simulink model "projeto_2016"  (R2016a)
settings: Solver=VariableStepAuto  StartTime=0.0  StopTime=t_sim  MaxStep=passo_integracao  RelTol=1e-3
values from neighbouring files (symbols this model uses):
  Kat = .3    (= 0.3)    [geracao.m]    (also in geracao_quadrado.m; parametros.m)
  x1_0 = -pi    (= -3.14159265359)    [geracao.m]    (also in geracao_quadrado.m = 0; parametros.m = 0)
  x2_0 = 0    [geracao.m]    (also in geracao_quadrado.m; parametros.m)
  x3_0 = 0    [geracao.m]    (also in geracao_quadrado.m; parametros.m)
  x4_0 = 0    [geracao.m]    (also in geracao_quadrado.m; parametros.m)
settings Model: Creator=ivanp_o3t94tg  LastModifiedBy=ivan_prog

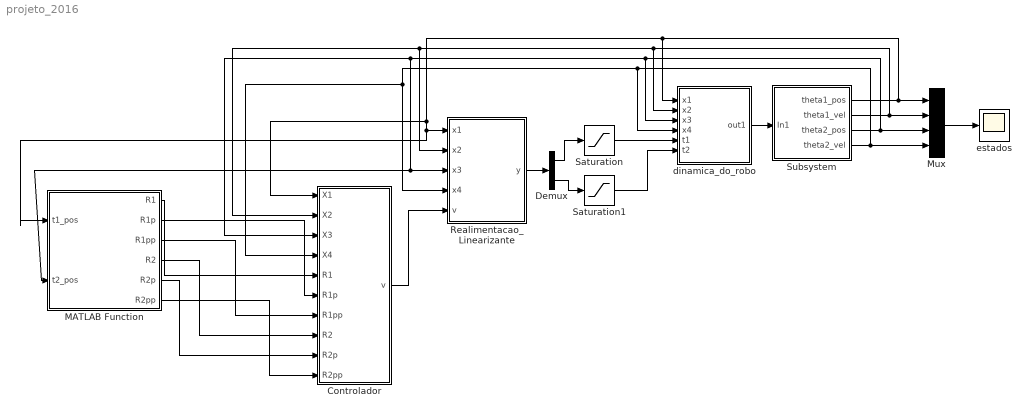
== system projeto_2016 ==
  Controlador : MATLAB Function  TreatAsAtomicUnit=on
  Demux : Demux  Outputs=2
  MATLAB Function : MATLAB Function  TreatAsAtomicUnit=on
  Mux : Mux
  Realimentacao_Linearizante : MATLAB Function  TreatAsAtomicUnit=on
  Saturation : Saturate  UpperLimit=100  LowerLimit=-100
  Saturation1 : Saturate  UpperLimit=100  LowerLimit=-100
  Subsystem : Subsystem
  dinamica_do_robo : MATLAB Function  TreatAsAtomicUnit=on
  estados : Scope
  wires:
  Mux/1 -> estados/1
  Subsystem/2(theta1_vel) -> Mux/2, dinamica_do_robo/2(x2), Controlador/2(X2), Realimentacao_Linearizante/2(x2)
  Subsystem/4(theta2_vel) -> dinamica_do_robo/4(x4), Realimentacao_Linearizante/4(x4), Controlador/4(X4), Mux/4
  Subsystem/1(theta1_pos) -> Mux/1, Controlador/1(X1), MATLAB Function/1(t1_pos), Realimentacao_Linearizante/1(x1), dinamica_do_robo/1(x1)
  Subsystem/3(theta2_pos) -> Mux/3, Controlador/3(X3), MATLAB Function/2(t2_pos), Realimentacao_Linearizante/3(x3), dinamica_do_robo/3(x3)
  dinamica_do_robo/1(out1) -> Subsystem/1(In1)
  Saturation/1 -> dinamica_do_robo/5(t1)
  Saturation1/1 -> dinamica_do_robo/6(t2)
  Realimentacao_Linearizante/1(y) -> Demux/1
  Demux/1 -> Saturation/1
  Demux/2 -> Saturation1/1
  Controlador/1(v) -> Realimentacao_Linearizante/5(v)
  MATLAB Function/1(R1) -> Controlador/5(R1)
  MATLAB Function/2(R1p) -> Controlador/6(R1p)
  MATLAB Function/3(R1pp) -> Controlador/7(R1pp)
  MATLAB Function/4(R2) -> Controlador/8(R2)
  MATLAB Function/5(R2p) -> Controlador/9(R2p)
  MATLAB Function/6(R2pp) -> Controlador/10(R2pp)

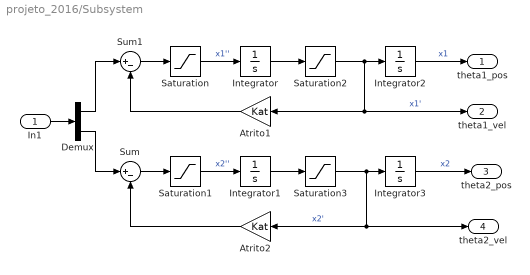
== system projeto_2016/Subsystem ==
  In1 : Inport
  Atrito1 : Gain  Gain=Kat
  Atrito2 : Gain  Gain=Kat
  Demux : Demux  Outputs=2
  Integrator : Integrator  InitialCondition=x2_0
  Integrator1 : Integrator  InitialCondition=x4_0
  Integrator2 : Integrator  InitialCondition=x1_0
  Integrator3 : Integrator  InitialCondition=x3_0
  Saturation{,1..3} (4 alike) : Saturate  UpperLimit=50  LowerLimit=-50
  Sum : Sum  Inputs=|+-
  Sum1 : Sum  Inputs=|+-
  theta1_pos : Outport
  theta1_vel : Outport  Port=2
  theta2_pos : Outport  Port=3
  theta2_vel : Outport  Port=4
  wires:
  Sum1/1 -> Saturation/1
  Saturation1/1 -> Integrator1/1  "x2''"
  Saturation2/1 -> theta1_vel/1, Atrito1/1, Integrator2/1  "x1'"
  In1/1 -> Demux/1
  Atrito2/1 -> Sum/2
  Saturation3/1 -> Atrito2/1, theta2_vel/1, Integrator3/1  "x2'"
  Integrator2/1 -> theta1_pos/1  "x1"
  Sum/1 -> Saturation1/1
  Integrator/1 -> Saturation2/1
  Demux/2 -> Sum/1
  Integrator3/1 -> theta2_pos/1  "x2"
  Demux/1 -> Sum1/1
  Saturation/1 -> Integrator/1  "x1''"
  Atrito1/1 -> Sum1/2
  Integrator1/1 -> Saturation3/1

== matlab function projeto_2016/Realimentacao_Linearizante ==
  data: x1 input; x2 input; x3 input; x4 input; v input; y output
function y = real_lin(x1,x2,x3,x4,v)

m1 = 2.2;
m2 = 2.2;
mp = 2;

L1 = 0.6;
L2 = 0.6;
l1 = 0.3;
l2 = 0.3;
I1 = 0.066;
I2 = 0.066;
g = 9.81;

% U = [t1;
%      t2];

m11 = I1+I2+m1*l1^2+(m2+mp)*L1^2+m2*(l2^2+L2^2)+2*L1*(m2*l2+mp*L2)*cos(x3);
m12 = I2+m2*l2^2+mp*L2^2+L1*(m2*l2+mp*L2)*cos(x3);
m21 = m12;
m22 = I2+m2^l2^2+mp*L2^2;

M = [m11 m12; 
     m21 m22];

g1 = (m1*l1+(m2+mp)*L1)*g*cos(x1)+(m2*l2+mp*L1)*g*cos(x1+x3);
g2 = (m2*l2+mp*L1)*g*cos(x1+x3);

h1 = -L1*(m2*l2+mp*L2)*sin(x3)*(2*x2*x4+x4^2)+g1;
h2 = L1*(m2*l2+mp*L2)*sin(x3)*x2^2+g2;

H = [h1;
     h2];

y = M*v+H;

== matlab function projeto_2016/dinamica_do_robo ==
  data: x1 input; x2 input; x3 input; x4 input; out1 output; t1 input; t2 input
function out1 = dinamica(x1,x2,x3,x4,t1,t2)
% x1 = theta1
% x2 = Dtheta1
% x3 = theta2
% x4 = Dtheta2
% t1 = torque1
% t2 = torque2

m1 = 2.2;
m2 = 2.2;
mp = 2;

L1 = 0.6;
L2 = 0.6;
l1 = 0.3;
l2 = 0.3;
I1 = 0.066;
I2 = 0.066;
g = 9.81;

U = [t1;
     t2];

m11 = I1+I2+m1*l1^2+(m2+mp)*L1^2+m2*(l2^2+L2^2)+2*L1*(m2*l2+mp*L2)*cos(x3);
m12 = I2+m2*l2^2+mp*L2^2+L1*(m2*l2+mp*L2)*cos(x3);
m21 = m12;
m22 = I2+m2^l2^2+mp*L2^2;

M = [m11 m12; 
     m21 m22];

g1 = (m1*l1+(m2+mp)*L1)*g*cos(x1)+(m2*l2+mp*L1)*g*cos(x1+x3);
g2 = (m2*l2+mp*L1)*g*cos(x1+x3);

h1 = -L1*(m2*l2+mp*L2)*sin(x3)*(2*x2*x4+x4^2)+g1;
h2 = L1*(m2*l2+mp*L2)*sin(x3)*x2^2+g2;

H = [h1;
     h2];
%out1 = inv(M)*(U-H);
out1 = M\(U-H);

end

== matlab function projeto_2016/Controlador ==
  data: X1 input; X2 input; X3 input; X4 input; R1 input; R1p input; R1pp input; v output; R2 input; R2p input; R2pp input
function v = ctrl(X1, X2, X3, X4, R1, R1p, R1pp, R2, R2p, R2pp)

r1pp = R1pp;
r1p  = R1p;
r1   = R1;

r2pp = R2pp;
r2p  = R2p;
r2   = R2;

theta1  = X1;
theta1p = X2;
theta2  = X3;
theta2p = X4;

e  = [r1-theta1;
      r2-theta2];
 
ep = [r1p-theta1p;
      r2p-theta2p];
  
t5_d = 0.1;
sd   = 4.8/t5_d;

kv11 = 2*sd;
kv22 = 2*sd;

kp11 = sd^2;
kp22 = sd^2;

kv = [kv11 0;
      0 kv22];

kp = [kp11 0;
      0 kp22];
  
v = [r1pp; r2pp]+kv*ep+kp*e;

== matlab function projeto_2016/MATLAB Function ==
  data: t1_pos input; R1 output; R1p output; R1pp output; R2 output; t2_pos input; R2p output; R2pp output
function [R1, R1p, R1pp, R2, R2p, R2pp]= ger_traj(t1_pos, t2_pos)

a = t1_pos;
b = t2_pos;

R1 = 0;
R1p = 0;
R1pp = 0;
R2 = 0;
R2p = 0;
R2pp = 0;
